simulink model "Model_silnika_PID_klasyk"  (R2024a)
settings: Solver=FixedStepAuto  StartTime=0.0  StopTime=czas_symulacji  RelTol=1e-3
undefined symbols (not defined in the file or in its folder): Kd, Ki, Kp
libraries: SignalEditorBlockLib x1
settings Model: Creator=kkucm  LastModifiedBy=krzysiek89
settings SolverCC: MaxConsecutiveMinStep=0.1
settings DebuggingCC: IgnoredZcDiagnostic=none
settings RTWCC: GPUComputeCapability=3.5

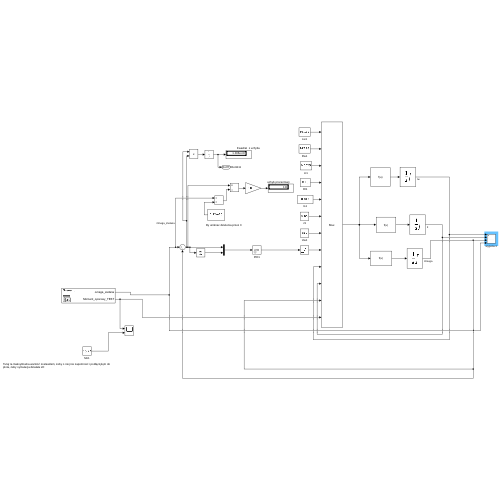
[thumbnail: Simulink's stored preview of the top-level diagram]
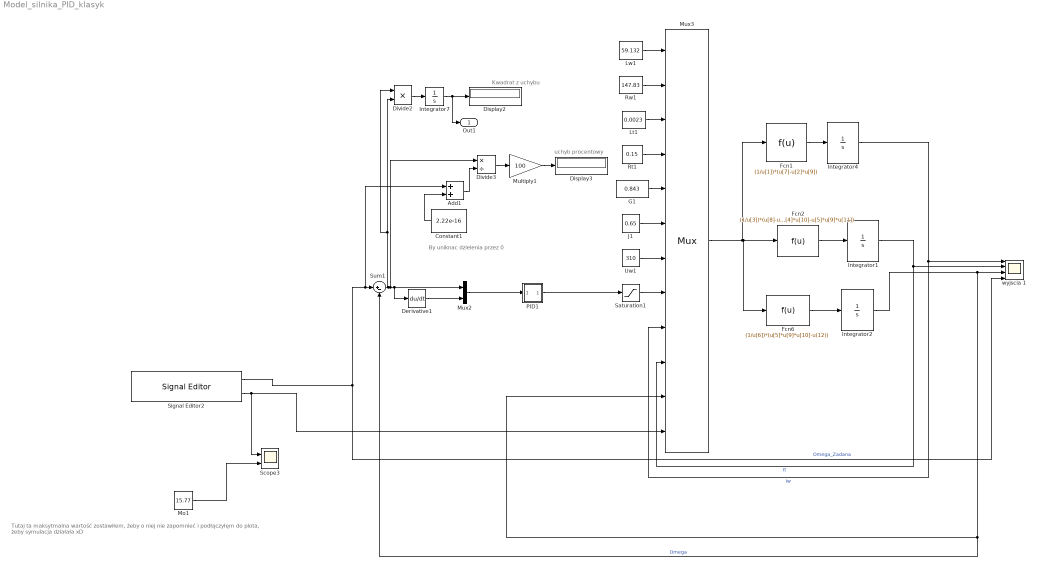
== system Model_silnika_PID_klasyk ==
  note: Kwadrat z uchybu
  note: Tutaj ta maksytmalna wartość zostawiłem, żeby o niej nie zapomnieć i podłączyłęm do plota, żeby symulacja działała xD
  note: uchyb procentowy
  note: By uniknac dzielenia przez 0
  Add1 : Sum
  Constant1 : Constant  Value=2.22e-16
  Derivative1 : Derivative
  Display2 : Display
  Display3 : Display
  Divide2 : Product  Inputs=**
  Divide3 : Product  Inputs=*/
  Fcn1 : Fcn  Expr=(1/u[1])*(u[7]-u[2]*u[9])
  Fcn2 : Fcn  Expr=(1/u[3])*(u[8]-u[4]*u[10]-u[5]*u[9]*u[11])
  Fcn6 : Fcn  Expr=(1/u[6])*(u[5]*u[9]*u[10]-u(12))
  G1 : Constant  Value=0.843  VectorParams1D=off
  Integrator1 : Integrator  InitialCondition=0.00001  LimitOutput=on  UpperSaturationLimit=1e3  LowerSaturationLimit=-1e3
  Integrator2 : Integrator  InitialCondition=0.00001  LimitOutput=on  UpperSaturationLimit=1e3  LowerSaturationLimit=-1e3
  Integrator4 : Integrator  InitialCondition=0.00001  LimitOutput=on  UpperSaturationLimit=1e3  LowerSaturationLimit=-1e3
  Integrator7 : Integrator  InitialCondition=0.00001  LowerSaturationLimit=1e-5
  J1 : Constant  Value=0.65
  Lt1 : Constant  Value=0.0023
  Lw1 : Constant  Value=59.132
  Mo1 : Constant  Value=15.77
  Multiply1 : Gain  Gain=100
  Mux2 : Mux  Inputs=2
  Mux3 : Mux  Inputs=12
  PID1 : Subsystem  mask(PID Controller){P=Kp, I=Ki, D=Kd}
      mask prompts: P "Proportional:"; I "Integral:"; D "Derivative:"
      mask help:
      | Enter expressions for proportional, integral, and derivative terms.
      | P+I/s+Ds
      mask Help: This block implements a PID controller where parameters are entered for the Proportional, Integral and Derivative terms. Unmask this block to see how it works. The derivative term is implemented using a true derivative block.
      mask Display: disp('PID')
  Rt1 : Constant  Value=0.15
  Rw1 : Constant  Value=147.83
  Saturation1 : Saturate  UpperLimit=528  LowerLimit=0
  Scope3 : Scope  NumInputPorts=2
  Signal Editor2 : SignalEditorBlockLib/Signal Editor  FileName=omega_zadana.mat  ActiveScenario=Scenario  ActiveSignal=omaga_zadana  IsBus=off  OutputBusObjectStr=Bus: BusObject  SampleTime=0  ZeroCross=off  OutputAfterFinalValue=Setting to zero  Unit=inherit  PreserveSignalName=on  ApplySigPropsToAllScenarios=on  ApplySigPropsToAllSignals=off
  Sum1 : Sum  Inputs=|+-
  Uw1 : Constant  Value=310
  wyjscia 1 : Scope  NumInputPorts=4
  Out1 : Outport  SignalName=Out1111
  wires:
  Sum1/1 -> Divide2/1, Divide2/2, Divide3/1, Derivative1/1, Mux2/1
  Fcn2/1 -> Integrator1/1
  Signal Editor2/2 -> Mux3/12, Scope3/1
  Mux2/1 -> PID1/1(In_1)
  Signal Editor2/1 -> wyjscia 1/4, Add1/1, Sum1/1  "Omega_Zadana"
  Lw1/1 -> Mux3/1
  Lt1/1 -> Mux3/3
  J1/1 -> Mux3/6
  Rw1/1 -> Mux3/2
  Fcn6/1 -> Integrator2/1
  Constant1/1 -> Add1/2
  Saturation1/1 -> Mux3/8
  G1/1 -> Mux3/5
  Integrator1/1 -> Mux3/10, wyjscia 1/2  "It"
  Rt1/1 -> Mux3/4
  Derivative1/1 -> Mux2/2
  Add1/1 -> Divide3/2
  Fcn1/1 -> Integrator4/1
  Integrator2/1 -> Mux3/11, Sum1/2, wyjscia 1/3  "Omega"
  Multiply1/1 -> Display3/1
  Mux3/1 -> Fcn1/1, Fcn6/1, Fcn2/1
  Divide3/1 -> Multiply1/1
  PID1/1(Out_1) -> Saturation1/1
  Integrator7/1 -> Out1/1, Display2/1
  Divide2/1 -> Integrator7/1
  Mo1/1 -> Scope3/2
  Uw1/1 -> Mux3/7
  Integrator4/1 -> Mux3/9, wyjscia 1/1  "Iw"

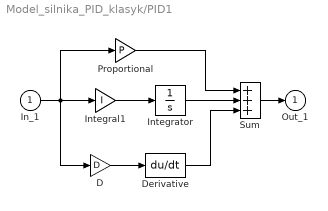
== system Model_silnika_PID_klasyk/PID1 ==
  In_1 : Inport
  D : Gain  Gain=D  SaturateOnIntegerOverflow=on  OutDataTypeStr=Inherit: Same as input  ParamDataTypeStr=Inherit: Same as input
  Derivative : Derivative
  Integral1 : Gain  Gain=I  SaturateOnIntegerOverflow=on  OutDataTypeStr=Inherit: Same as input  ParamDataTypeStr=Inherit: Same as input
  Integrator : Integrator  LimitOutput=on  UpperSaturationLimit=0.3  LowerSaturationLimit=-0.3
  Proportional : Gain  Gain=P  SaturateOnIntegerOverflow=on  OutDataTypeStr=Inherit: Same as input  ParamDataTypeStr=Inherit: Same as input
  Sum : Sum  Inputs=+++  InputSameDT=on  SaturateOnIntegerOverflow=on  OutDataTypeStr=Inherit: Same as first input
  Out_1 : Outport  InitialOutput=0
  wires:
  Proportional/1 -> Sum/1
  Integrator/1 -> Sum/2
  Derivative/1 -> Sum/3
  In_1/1 -> Proportional/1, Integral1/1, D/1
  Sum/1 -> Out_1/1
  D/1 -> Derivative/1
  Integral1/1 -> Integrator/1
